simulink model "task4"  (R2024a)
settings: Solver=VariableStepAuto  StartTime=0.0  StopTime=10.0  MaxStep=0.001  RelTol=1e-3
undefined symbols (not defined in the file): A, Abar, B, Bbar, Bfbar, C, D, Df, Gamma_f, Kw, Kx, L, wf0, x0_bar, x0_hat, Yf
settings Model: Creator=sizgr  LastModifiedBy=sizgr

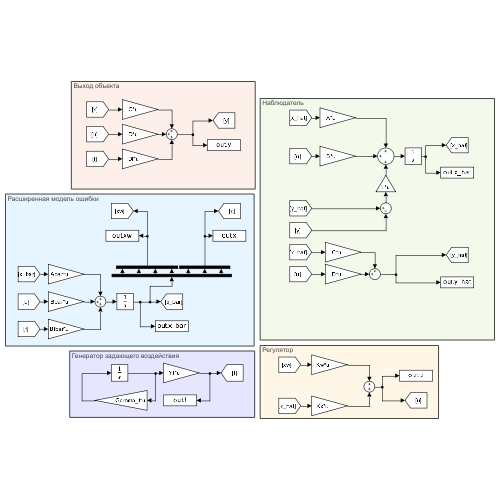
[thumbnail: Simulink's stored preview of the top-level diagram]
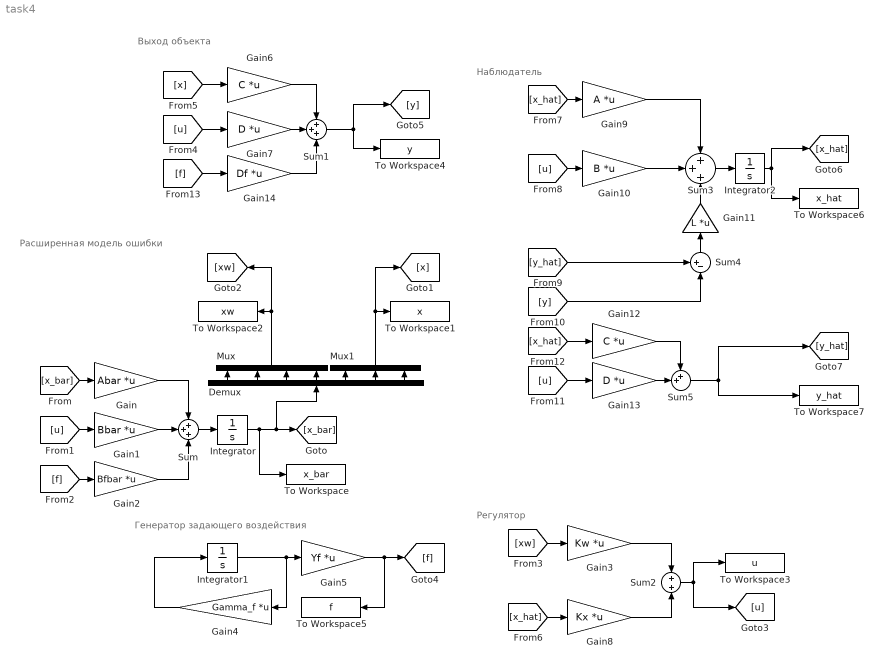
== system task4 ==
  note: Наблюдатель
  note: Регулятор
  note: Выход объекта
  note: Расширенная модель ошибки
  note: Генератор задающего воздействия
  Demux : Demux  Outputs=7
  Gain : Gain  Gain=Abar  Multiplication=Matrix(K*u)
  Gain1 : Gain  Gain=Bbar  Multiplication=Matrix(K*u)
  Gain10 : Gain  Gain=B  Multiplication=Matrix(K*u)
  Gain11 : Gain  Gain=L  Multiplication=Matrix(K*u)
  Gain12 : Gain  Gain=C  Multiplication=Matrix(K*u)
  Gain13 : Gain  Gain=D  Multiplication=Matrix(K*u)
  Gain14 : Gain  Gain=Df  Multiplication=Matrix(K*u)
  Gain2 : Gain  Gain=Bfbar  Multiplication=Matrix(K*u)
  Gain3 : Gain  Gain=Kw  Multiplication=Matrix(K*u)
  Gain4 : Gain  Gain=Gamma_f  Multiplication=Matrix(K*u)
  Gain5 : Gain  Gain=Yf  Multiplication=Matrix(K*u)
  Gain6 : Gain  Gain=C  Multiplication=Matrix(K*u)
  Gain7 : Gain  Gain=D  Multiplication=Matrix(K*u)
  Gain8 : Gain  Gain=Kx  Multiplication=Matrix(K*u)
  Gain9 : Gain  Gain=A  Multiplication=Matrix(K*u)
  Integrator : Integrator  InitialCondition=x0_bar
  Integrator1 : Integrator  InitialCondition=wf0
  Integrator2 : Integrator  InitialCondition=x0_hat
  Mux : Mux
  Mux1 : Mux  Inputs=3
  Sum : Sum  Inputs=+++
  Sum1 : Sum  Inputs=+++
  Sum2 : Sum  Inputs=+|+
  Sum3 : Sum  Inputs=+++
  Sum4 : Sum  Inputs=+-|
  Sum5 : Sum  Inputs=++|
  To Workspace : ToWorkspace  VariableName=x_bar  SaveFormat=Timeseries  SampleTime=-1
  To Workspace1 : ToWorkspace  VariableName=x  SaveFormat=Timeseries  SampleTime=-1
  To Workspace2 : ToWorkspace  VariableName=xw  SaveFormat=Timeseries  SampleTime=-1
  To Workspace3 : ToWorkspace  VariableName=u  SaveFormat=Timeseries  SampleTime=-1
  To Workspace4 : ToWorkspace  VariableName=y  SaveFormat=Timeseries  SampleTime=-1
  To Workspace5 : ToWorkspace  VariableName=f  SaveFormat=Timeseries  SampleTime=-1
  To Workspace6 : ToWorkspace  VariableName=x_hat  SaveFormat=Timeseries  SampleTime=-1
  To Workspace7 : ToWorkspace  VariableName=y_hat  SaveFormat=Timeseries  SampleTime=-1
  wires:
  Sum2/1 -> To Workspace3/1, [u]
  [xw] -> Gain3/1
  [x_hat] -> Gain8/1
  Gain3/1 -> Sum2/1
  Gain8/1 -> Sum2/2
  [x_hat] -> Gain9/1
  Gain10/1 -> Sum3/2
  Integrator2/1 -> To Workspace6/1, [x_hat]
  Sum3/1 -> Integrator2/1
  Gain9/1 -> Sum3/1
  [u] -> Gain10/1
  [y_hat] -> Sum4/1
  [y] -> Sum4/2
  Sum4/1 -> Gain11/1
  [u] -> Gain13/1
  Gain12/1 -> Sum5/1
  Gain13/1 -> Sum5/2
  Sum5/1 -> To Workspace7/1, [y_hat]
  [x_hat] -> Gain12/1
  Demux/3 -> Mux/3
  Demux/7 -> Mux1/3
  Demux/4 -> Mux/4
  Demux/5 -> Mux1/1
  [x_bar] -> Gain/1
  [x] -> Gain6/1
  [u] -> Gain1/1
  Demux/6 -> Mux1/2
  Mux1/1 -> [x], To Workspace1/1
  Integrator/1 -> Demux/1, [x_bar], To Workspace/1
  Demux/1 -> Mux/1
  Mux/1 -> To Workspace2/1, [xw]
  Gain14/1 -> Sum1/3
  Sum1/1 -> To Workspace4/1, [y]
  Demux/2 -> Mux/2
  Gain6/1 -> Sum1/1
  Gain7/1 -> Sum1/2
  [u] -> Gain7/1
  [f] -> Gain14/1
  Gain/1 -> Sum/1
  Gain1/1 -> Sum/2
  Gain2/1 -> Sum/3
  Sum/1 -> Integrator/1
  [f] -> Gain2/1
  Gain5/1 -> [f], To Workspace5/1
  Gain4/1 -> Integrator1/1
  Integrator1/1 -> Gain5/1, Gain4/1
  Gain11/1 -> Sum3/3
